simulink model "SecRwRtStLgrstUpwdDnwdIsPosChk"  (R2024b)
settings: Solver=FixedStepDiscrete  StartTime=0.0  StopTime=10.0  FixedStep=0.01  RelTol=1e-3
undefined symbols (not defined in the file or in its folder): KeSMSuSecRwStLegrestUpwdDwnwdPosDelta_Val, KeSMSuSecRwStLegrestUpwdDwnwdPosTolr_Val
libraries: StIsPosChkLib x19, simulink x8
(part 1 of 2)
settings Model: Creator=sn2xws  LastModifiedBy=sn55gm
settings Model: ModifiedHistory=|
  | 2023.8.1 V2.0.0 CR421790 增加模式21-26
  | 2024.7.8 V3.0.0 557模式流程V1.9
  | 2024.8.15 V3.0.1 智享模式需要计算目标位置，不能直接判断到位置，posalready赋值0
  | 2024.9.5 V3.0.2 新增Md56，注释不用的模式
  | 2024.10.14 V3.0.3 新增Md57 Md58
  | 2024.11.27 V3.0.4 Md57运行时不能直接判断到位置
  | 25.7.7 V3.13.0 新增Md61 Md62 md30 md31
  | 25.7.15 Md30secstage2done_Val_read增加接口作为目标位置判断
settings SolverCC: AlgebraicLoopSolver=TrustRegion
settings DataIOCC: SaveFormat=StructureWithTime  ReturnWorkspaceOutputs=off
settings OptimizationCC: DefaultParameterBehavior=Inlined  EnhancedBackFolding=on  PassReuseOutputArgsAs=Individual arguments  ZeroExternalMemoryAtStartup=off  ZeroInternalMemoryAtStartup=off  OptimizeBlockOrder=speed  DifferentSizesBufferReuse=on  OptimizationCustomize=off  EfficientTunableParamExpr=on
settings DebuggingCC: ParameterTunabilityLossMsg=error  UnconnectedInputMsg=warning  UnconnectedOutputMsg=warning  UnconnectedLineMsg=warning  ArithmeticOperatorsInVariantConditions=warning
settings ModelReferenceCC: EnableRefExpFcnMdlSchedulingChecks=on  ModelReferenceNumInstancesAllowed=Single
settings SFSimCC: MATLABDynamicMemAlloc=off  CustomCodeUndefinedFunction=UseInterfaceOnly
settings RTWCC: Description=AUTOSAR  SystemTargetFile=autosar.tlc  GenCodeOnly=on  TemplateMakefile=ert_default_tmf  GenerateReport=on  IncludeHyperlinkInReport=on  LaunchReport=on  DataTypeReplacement=CDataTypesFixedWidth  GenerateTraceInfo=on  GenerateTraceReport=on  GenerateTraceReportSl=on  GenerateTraceReportSf=on  GenerateTraceReportEml=on  GPUComputeCapability=3.5
settings CodeAppCC: ForceParamTrailComments=on  IgnoreCustomStorageClasses=off  OperatorAnnotations=on  SimulinkDataObjDesc=on  SFDataObjDesc=on  InsertBlockDesc=on
settings STFCustomTargetCC: TargetLangStandard=C99 (ISO)  MultiwordLength=256  ParMdlRefBuildCompliant=on  CompOptLevelCompliant=on  IncludeMdlTerminateFcn=off  CombineOutputUpdateFcns=on  SuppressErrorStatus=on  ERTCustomFileBanners=on  SupportNonFinite=off  SupportComplex=off  SupportContinuousTime=off  SupportNonInlinedSFcns=off  RemoveResetFunc=on  MATLABClassNameForMDSCustomization=Simulink.SoftwareTarget.ERTCustomization  AutosarCompliant=on  UseToolchainInfoCompliant=on  LookupTableObjectStructAxisOrder=2,1,3,4,...  LUTObjectStructOrderEvenSpacing=Size,Table,Breakpoints  SystemTargetFile=autosar.tlc
settings ERTTargetCC: TargetLangStandard=C99 (ISO)  ConcurrentExecutionCompliant=off  IncludeMdlTerminateFcn=off  SuppressErrorStatus=on  SupportNonFinite=off  SupportComplex=off  ModelStepFunctionPrototypeControlCompliant=off  CPPClassGenCompliant=off  AutosarCompliant=on  LookupTableObjectStructAxisOrder=2,1,3,4,...  LUTObjectStructOrderEvenSpacing=Size,Table,Breakpoints  ERTCustomFileTemplate=example_file_process.tlc  ERTFilePackagingFormat=Compact  BooleanTrueId=TRUE  BooleanFalseId=FALSE  DynamicArrayContainerType=coder::array

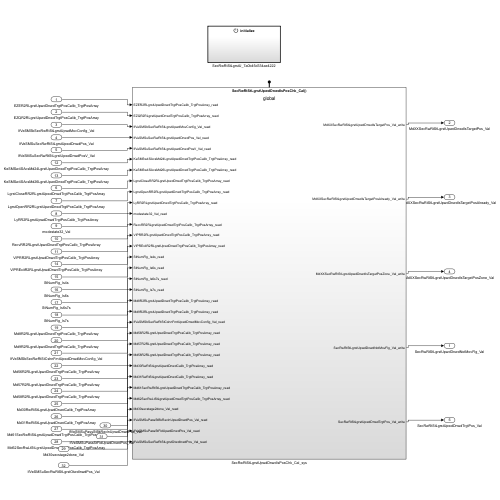
[thumbnail: Simulink's stored preview of the top-level diagram]
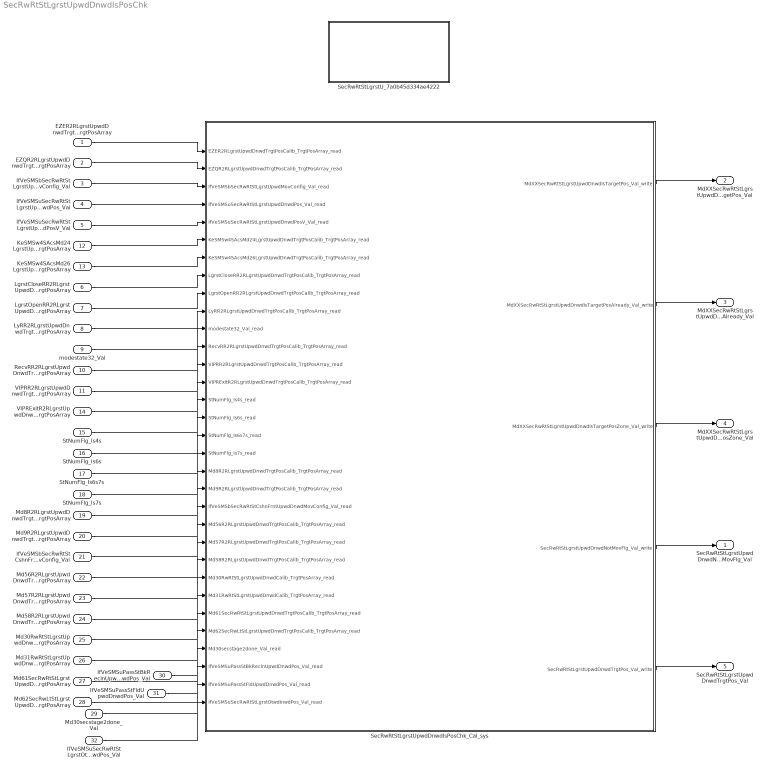
== system SecRwRtStLgrstUpwdDnwdIsPosChk ==
  EZER2RLgrstUpwdDnwdTrgtPosCalib_TrgtPosArray : Inport  Description=|  OutDataTypeStr=uint16  PortDimensions=3
      | 0:Pos
      | 1:Max
      | 2:Min
  EZQR2RLgrstUpwdDnwdTrgtPosCalib_TrgtPosArray : Inport  Description=|  Port=2  OutDataTypeStr=uint16  PortDimensions=3
      | 0:Pos
      | 1:Max
      | 2:Min
  IfVeSMSbSecRwRtStLgrstUpwdMovConfig_Val : Inport  Port=3  OutDataTypeStr=boolean  PortDimensions=1
  IfVeSMSuSecRwRtStLgrstUpwdDnwdPos_Val : Inport  Port=4  OutDataTypeStr=uint16  PortDimensions=1
  IfVeSMSuSecRwRtStLgrstUpwdDnwdPosV_Val : Inport  Port=5  OutDataTypeStr=boolean  PortDimensions=1
  LgrstCloseRR2RLgrstUpwdDnwdTrgtPosCalib_TrgtPosArray : Inport  Description=|  Port=6  OutDataTypeStr=uint16  PortDimensions=3
      | 0:Pos
      | 1:Max
      | 2:Min
  LgrstOpenRR2RLgrstUpwdDnwdTrgtPosCalib_TrgtPosArray : Inport  Description=|  Port=7  OutDataTypeStr=uint16  PortDimensions=3
      | 0:Pos
      | 1:Max
      | 2:Min
  LyRR2RLgrstUpwdDnwdTrgtPosCalib_TrgtPosArray : Inport  Description=|  Port=8  OutDataTypeStr=uint16  PortDimensions=3
      | 0:Pos
      | 1:Max
      | 2:Min
  modestate32_Val : Inport  Port=9  OutDataTypeStr=uint32  PortDimensions=1
  RecvRR2RLgrstUpwdDnwdTrgtPosCalib_TrgtPosArray : Inport  Description=|  Port=10  OutDataTypeStr=uint16  PortDimensions=3
      | 0:Pos
      | 1:Max
      | 2:Min
  VIPRR2RLgrstUpwdDnwdTrgtPosCalib_TrgtPosArray : Inport  Description=|  Port=11  OutDataTypeStr=uint16  PortDimensions=3
      | 0:Pos
      | 1:Max
      | 2:Min
  KeSMSw4SAcsMd24LgrstUpwdDnwdTrgtPosCalib_TrgtPosArray : Inport  Description=|  Port=12  OutDataTypeStr=uint16  PortDimensions=3
      | 0:Pos
      | 1:Max
      | 2:Min
  KeSMSw4SAcsMd26LgrstUpwdDnwdTrgtPosCalib_TrgtPosArray : Inport  Description=|  Port=13  OutDataTypeStr=uint16  PortDimensions=3
      | 0:Pos
      | 1:Max
      | 2:Min
  VIPRExitR2RLgrstUpwdDnwdTrgtPosCalib_TrgtPosArray : Inport  Description=|  Port=14  OutDataTypeStr=uint16  PortDimensions=3
      | 0:Pos
      | 1:Max
      | 2:Min
  StNumFlg_Is4s : Inport  Port=15  OutDataTypeStr=boolean  PortDimensions=1
  StNumFlg_Is6s : Inport  Port=16  OutDataTypeStr=boolean  PortDimensions=1
  StNumFlg_Is6s7s : Inport  Port=17  OutDataTypeStr=boolean  PortDimensions=1
  StNumFlg_Is7s : Inport  Port=18  OutDataTypeStr=boolean  PortDimensions=1
  Md8R2RLgrstUpwdDnwdTrgtPosCalib_TrgtPosArray : Inport  Description=|  Port=19  OutDataTypeStr=uint16  PortDimensions=3
      | 0:Pos
      | 1:Max
      | 2:Min
  Md9R2RLgrstUpwdDnwdTrgtPosCalib_TrgtPosArray : Inport  Description=|  Port=20  OutDataTypeStr=uint16  PortDimensions=3
      | 0:Pos
      | 1:Max
      | 2:Min
  IfVeSMSbSecRwRtStCshnFrntUpwdDnwdMovConfig_Val : Inport  Port=21  OutDataTypeStr=boolean  PortDimensions=1
  Md56R2RLgrstUpwdDnwdTrgtPosCalib_TrgtPosArray : Inport  Description=|  Port=22  OutDataTypeStr=uint16  PortDimensions=3
      | 0:Pos
      | 1:Max
      | 2:Min
  Md57R2RLgrstUpwdDnwdTrgtPosCalib_TrgtPosArray : Inport  Description=|  Port=23  OutDataTypeStr=uint16  PortDimensions=3
      | 0:Pos
      | 1:Max
      | 2:Min
  Md58R2RLgrstUpwdDnwdTrgtPosCalib_TrgtPosArray : Inport  Description=|  Port=24  OutDataTypeStr=uint16  PortDimensions=3
      | 0:Pos
      | 1:Max
      | 2:Min
  Md30RwRtStLgrstUpwdDnwdCalib_TrgtPosArray : Inport  Description=|  Port=25  OutDataTypeStr=uint16  PortDimensions=3
      | 0:Pos
      | 1:Max
      | 2:Min
  Md31RwRtStLgrstUpwdDnwdCalib_TrgtPosArray : Inport  Description=|  Port=26  OutDataTypeStr=uint16  PortDimensions=3
      | 0:Pos
      | 1:Max
      | 2:Min
  Md61SecRwRtStLgrstUpwdDnwdTrgtPosCalib_TrgtPosArray : Inport  Description=|  Port=27  OutDataTypeStr=uint16  PortDimensions=3
      | 0:Pos
      | 1:Max
      | 2:Min
  Md62SecRwLtStLgrstUpwdDnwdTrgtPosCalib_TrgtPosArray : Inport  Description=|  Port=28  OutDataTypeStr=uint16  PortDimensions=3
      | 0:Pos
      | 1:Max
      | 2:Min
  Md30secstage2done_Val : Inport  Port=29  OutDataTypeStr=uint8  PortDimensions=1
  IfVeSMSuPassStBkReclnUpwdDnwdPos_Val : Inport  Port=30  OutDataTypeStr=uint16  PortDimensions=1
  IfVeSMSuPassStFldUpwdDnwdPos_Val : Inport  Port=31  OutDataTypeStr=uint16  PortDimensions=1
  IfVeSMSuSecRwRtStLgrstOtwdInwdPos_Val : Inport  Port=32  OutDataTypeStr=uint16  PortDimensions=1
  SecRwRtStLgrstU_7a0b45d334ae4222 : Subsystem
  SecRwRtStLgrstUpwdDnwdIsPosChk_Cal_sys : Subsystem
  SecRwRtStLgrstUpwdDnwdNotMovFlg_Val : Outport  OutDataTypeStr=boolean  PortDimensions=1  VectorParamsAs1DForOutWhenUnconnected=off
  MdXXSecRwRtStLgrstUpwdDnwdIsTargetPos_Val : Outport  Port=2  OutDataTypeStr=uint32  PortDimensions=1  VectorParamsAs1DForOutWhenUnconnected=off
  MdXXSecRwRtStLgrstUpwdDnwdIsTargetPosAlready_Val : Outport  Port=3  OutDataTypeStr=uint32  PortDimensions=1  VectorParamsAs1DForOutWhenUnconnected=off
  MdXXSecRwRtStLgrstUpwdDnwdIsTargetPosZone_Val : Outport  Port=4  OutDataTypeStr=uint32  PortDimensions=1  VectorParamsAs1DForOutWhenUnconnected=off
  SecRwRtStLgrstUpwdDnwdTrgtPos_Val : Outport  Port=5  OutDataTypeStr=uint16  PortDimensions=1  VectorParamsAs1DForOutWhenUnconnected=off
  wires:
  EZER2RLgrstUpwdDnwdTrgtPosCalib_TrgtPosArray/1 -> SecRwRtStLgrstUpwdDnwdIsPosChk_Cal_sys/1(EZER2RLgrstUpwdDnwdTrgtPosCalib_TrgtPosArray_read)
  EZQR2RLgrstUpwdDnwdTrgtPosCalib_TrgtPosArray/1 -> SecRwRtStLgrstUpwdDnwdIsPosChk_Cal_sys/2(EZQR2RLgrstUpwdDnwdTrgtPosCalib_TrgtPosArray_read)
  IfVeSMSbSecRwRtStLgrstUpwdMovConfig_Val/1 -> SecRwRtStLgrstUpwdDnwdIsPosChk_Cal_sys/3(IfVeSMSbSecRwRtStLgrstUpwdMovConfig_Val_read)
  IfVeSMSuSecRwRtStLgrstUpwdDnwdPos_Val/1 -> SecRwRtStLgrstUpwdDnwdIsPosChk_Cal_sys/4(IfVeSMSuSecRwRtStLgrstUpwdDnwdPos_Val_read)
  IfVeSMSuSecRwRtStLgrstUpwdDnwdPosV_Val/1 -> SecRwRtStLgrstUpwdDnwdIsPosChk_Cal_sys/5(IfVeSMSuSecRwRtStLgrstUpwdDnwdPosV_Val_read)
  LgrstCloseRR2RLgrstUpwdDnwdTrgtPosCalib_TrgtPosArray/1 -> SecRwRtStLgrstUpwdDnwdIsPosChk_Cal_sys/8(LgrstCloseRR2RLgrstUpwdDnwdTrgtPosCalib_TrgtPosArray_read)
  LgrstOpenRR2RLgrstUpwdDnwdTrgtPosCalib_TrgtPosArray/1 -> SecRwRtStLgrstUpwdDnwdIsPosChk_Cal_sys/9(LgrstOpenRR2RLgrstUpwdDnwdTrgtPosCalib_TrgtPosArray_read)
  LyRR2RLgrstUpwdDnwdTrgtPosCalib_TrgtPosArray/1 -> SecRwRtStLgrstUpwdDnwdIsPosChk_Cal_sys/10(LyRR2RLgrstUpwdDnwdTrgtPosCalib_TrgtPosArray_read)
  modestate32_Val/1 -> SecRwRtStLgrstUpwdDnwdIsPosChk_Cal_sys/11(modestate32_Val_read)
  RecvRR2RLgrstUpwdDnwdTrgtPosCalib_TrgtPosArray/1 -> SecRwRtStLgrstUpwdDnwdIsPosChk_Cal_sys/12(RecvRR2RLgrstUpwdDnwdTrgtPosCalib_TrgtPosArray_read)
  VIPRR2RLgrstUpwdDnwdTrgtPosCalib_TrgtPosArray/1 -> SecRwRtStLgrstUpwdDnwdIsPosChk_Cal_sys/13(VIPRR2RLgrstUpwdDnwdTrgtPosCalib_TrgtPosArray_read)
  SecRwRtStLgrstUpwdDnwdIsPosChk_Cal_sys/1(MdXXSecRwRtStLgrstUpwdDnwdIsTargetPos_Val_write) -> MdXXSecRwRtStLgrstUpwdDnwdIsTargetPos_Val/1
  SecRwRtStLgrstUpwdDnwdIsPosChk_Cal_sys/2(MdXXSecRwRtStLgrstUpwdDnwdIsTargetPosAlready_Val_write) -> MdXXSecRwRtStLgrstUpwdDnwdIsTargetPosAlready_Val/1
  SecRwRtStLgrstUpwdDnwdIsPosChk_Cal_sys/3(MdXXSecRwRtStLgrstUpwdDnwdIsTargetPosZone_Val_write) -> MdXXSecRwRtStLgrstUpwdDnwdIsTargetPosZone_Val/1
  SecRwRtStLgrstUpwdDnwdIsPosChk_Cal_sys/4(SecRwRtStLgrstUpwdDnwdNotMovFlg_Val_write) -> SecRwRtStLgrstUpwdDnwdNotMovFlg_Val/1
  SecRwRtStLgrstUpwdDnwdIsPosChk_Cal_sys/5(SecRwRtStLgrstUpwdDnwdTrgtPos_Val_write) -> SecRwRtStLgrstUpwdDnwdTrgtPos_Val/1
  KeSMSw4SAcsMd24LgrstUpwdDnwdTrgtPosCalib_TrgtPosArray/1 -> SecRwRtStLgrstUpwdDnwdIsPosChk_Cal_sys/6(KeSMSw4SAcsMd24LgrstUpwdDnwdTrgtPosCalib_TrgtPosArray_read)
  KeSMSw4SAcsMd26LgrstUpwdDnwdTrgtPosCalib_TrgtPosArray/1 -> SecRwRtStLgrstUpwdDnwdIsPosChk_Cal_sys/7(KeSMSw4SAcsMd26LgrstUpwdDnwdTrgtPosCalib_TrgtPosArray_read)
  VIPRExitR2RLgrstUpwdDnwdTrgtPosCalib_TrgtPosArray/1 -> SecRwRtStLgrstUpwdDnwdIsPosChk_Cal_sys/14(VIPRExitR2RLgrstUpwdDnwdTrgtPosCalib_TrgtPosArray_read)
  StNumFlg_Is4s/1 -> SecRwRtStLgrstUpwdDnwdIsPosChk_Cal_sys/15(StNumFlg_Is4s_read)
  StNumFlg_Is6s/1 -> SecRwRtStLgrstUpwdDnwdIsPosChk_Cal_sys/16(StNumFlg_Is6s_read)
  StNumFlg_Is6s7s/1 -> SecRwRtStLgrstUpwdDnwdIsPosChk_Cal_sys/17(StNumFlg_Is6s7s_read)
  StNumFlg_Is7s/1 -> SecRwRtStLgrstUpwdDnwdIsPosChk_Cal_sys/18(StNumFlg_Is7s_read)
  Md8R2RLgrstUpwdDnwdTrgtPosCalib_TrgtPosArray/1 -> SecRwRtStLgrstUpwdDnwdIsPosChk_Cal_sys/19(Md8R2RLgrstUpwdDnwdTrgtPosCalib_TrgtPosArray_read)
  Md9R2RLgrstUpwdDnwdTrgtPosCalib_TrgtPosArray/1 -> SecRwRtStLgrstUpwdDnwdIsPosChk_Cal_sys/20(Md9R2RLgrstUpwdDnwdTrgtPosCalib_TrgtPosArray_read)
  IfVeSMSbSecRwRtStCshnFrntUpwdDnwdMovConfig_Val/1 -> SecRwRtStLgrstUpwdDnwdIsPosChk_Cal_sys/21(IfVeSMSbSecRwRtStCshnFrntUpwdDnwdMovConfig_Val_read)
  Md56R2RLgrstUpwdDnwdTrgtPosCalib_TrgtPosArray/1 -> SecRwRtStLgrstUpwdDnwdIsPosChk_Cal_sys/22(Md56R2RLgrstUpwdDnwdTrgtPosCalib_TrgtPosArray_read)
  Md57R2RLgrstUpwdDnwdTrgtPosCalib_TrgtPosArray/1 -> SecRwRtStLgrstUpwdDnwdIsPosChk_Cal_sys/23(Md57R2RLgrstUpwdDnwdTrgtPosCalib_TrgtPosArray_read)
  Md58R2RLgrstUpwdDnwdTrgtPosCalib_TrgtPosArray/1 -> SecRwRtStLgrstUpwdDnwdIsPosChk_Cal_sys/24(Md58R2RLgrstUpwdDnwdTrgtPosCalib_TrgtPosArray_read)
  Md30RwRtStLgrstUpwdDnwdCalib_TrgtPosArray/1 -> SecRwRtStLgrstUpwdDnwdIsPosChk_Cal_sys/25(Md30RwRtStLgrstUpwdDnwdCalib_TrgtPosArray_read)
  Md31RwRtStLgrstUpwdDnwdCalib_TrgtPosArray/1 -> SecRwRtStLgrstUpwdDnwdIsPosChk_Cal_sys/26(Md31RwRtStLgrstUpwdDnwdCalib_TrgtPosArray_read)
  Md61SecRwRtStLgrstUpwdDnwdTrgtPosCalib_TrgtPosArray/1 -> SecRwRtStLgrstUpwdDnwdIsPosChk_Cal_sys/27(Md61SecRwRtStLgrstUpwdDnwdTrgtPosCalib_TrgtPosArray_read)
  Md62SecRwLtStLgrstUpwdDnwdTrgtPosCalib_TrgtPosArray/1 -> SecRwRtStLgrstUpwdDnwdIsPosChk_Cal_sys/28(Md62SecRwLtStLgrstUpwdDnwdTrgtPosCalib_TrgtPosArray_read)
  Md30secstage2done_Val/1 -> SecRwRtStLgrstUpwdDnwdIsPosChk_Cal_sys/29(Md30secstage2done_Val_read)
  IfVeSMSuPassStBkReclnUpwdDnwdPos_Val/1 -> SecRwRtStLgrstUpwdDnwdIsPosChk_Cal_sys/30(IfVeSMSuPassStBkReclnUpwdDnwdPos_Val_read)
  IfVeSMSuPassStFldUpwdDnwdPos_Val/1 -> SecRwRtStLgrstUpwdDnwdIsPosChk_Cal_sys/31(IfVeSMSuPassStFldUpwdDnwdPos_Val_read)
  IfVeSMSuSecRwRtStLgrstOtwdInwdPos_Val/1 -> SecRwRtStLgrstUpwdDnwdIsPosChk_Cal_sys/32(IfVeSMSuSecRwRtStLgrstOtwdInwdPos_Val_read)

== system SecRwRtStLgrstUpwdDnwdIsPosChk/SecRwRtStLgrstU_7a0b45d334ae4222 ==
  note: Added blocks
  note: Added blocks
  Event Listener : EventListener  EventName=reset
  PA_KeSMSuSecRwStLegrestUpwdDwnwdPosDelta_Val : Constant  Value=KeSMSuSecRwStLegrestUpwdDwnwdPosDelta_Val
  PA_KeSMSuSecRwStLegrestUpwdDwnwdPosTolr_Val : Constant  Value=KeSMSuSecRwStLegrestUpwdDwnwdPosTolr_Val
  Terminator_1 : Terminator
  Terminator_2 : Terminator
  wires:
  PA_KeSMSuSecRwStLegrestUpwdDwnwdPosDelta_Val/1 -> Terminator_1/1
  PA_KeSMSuSecRwStLegrestUpwdDwnwdPosTolr_Val/1 -> Terminator_2/1

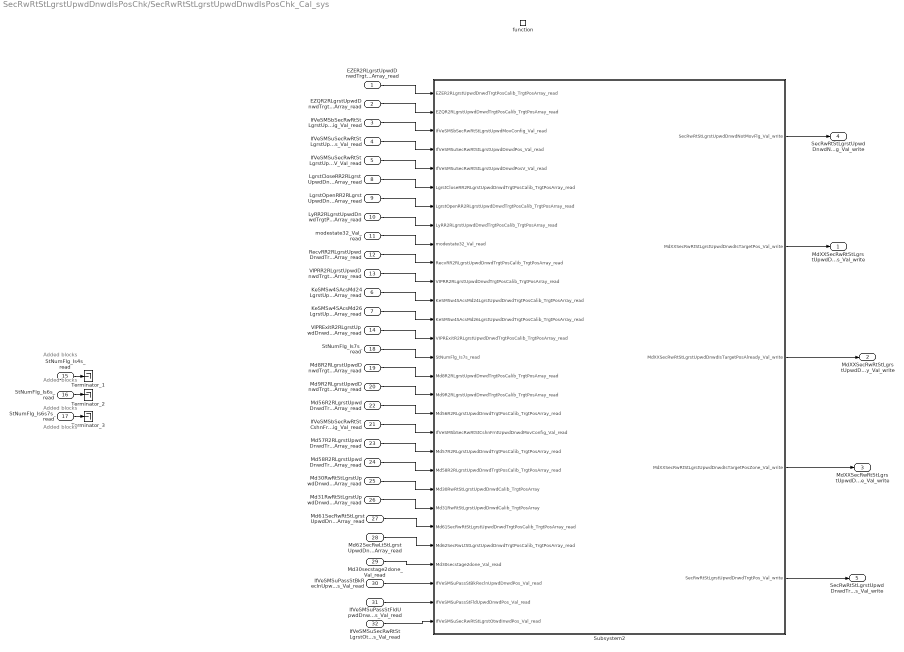
== system SecRwRtStLgrstUpwdDnwdIsPosChk/SecRwRtStLgrstUpwdDnwdIsPosChk_Cal_sys ==
  note: Added blocks
  note: Added blocks
  note: Added blocks
  note: Added blocks
  EZER2RLgrstUpwdDnwdTrgtPosCalib_TrgtPosArray_read : Inport
  EZQR2RLgrstUpwdDnwdTrgtPosCalib_TrgtPosArray_read : Inport  Port=2
  IfVeSMSbSecRwRtStLgrstUpwdMovConfig_Val_read : Inport  Port=3
  IfVeSMSuSecRwRtStLgrstUpwdDnwdPos_Val_read : Inport  Port=4
  IfVeSMSuSecRwRtStLgrstUpwdDnwdPosV_Val_read : Inport  Port=5
  KeSMSw4SAcsMd24LgrstUpwdDnwdTrgtPosCalib_TrgtPosArray_read : Inport  Port=6
  KeSMSw4SAcsMd26LgrstUpwdDnwdTrgtPosCalib_TrgtPosArray_read : Inport  Port=7
  LgrstCloseRR2RLgrstUpwdDnwdTrgtPosCalib_TrgtPosArray_read : Inport  Port=8
  LgrstOpenRR2RLgrstUpwdDnwdTrgtPosCalib_TrgtPosArray_read : Inport  Port=9
  LyRR2RLgrstUpwdDnwdTrgtPosCalib_TrgtPosArray_read : Inport  Port=10
  modestate32_Val_read : Inport  Port=11
  RecvRR2RLgrstUpwdDnwdTrgtPosCalib_TrgtPosArray_read : Inport  Port=12
  VIPRR2RLgrstUpwdDnwdTrgtPosCalib_TrgtPosArray_read : Inport  Port=13
  VIPRExitR2RLgrstUpwdDnwdTrgtPosCalib_TrgtPosArray_read : Inport  Port=14
  StNumFlg_Is4s_read : Inport  Port=15
  StNumFlg_Is6s_read : Inport  Port=16
  StNumFlg_Is6s7s_read : Inport  Port=17
  StNumFlg_Is7s_read : Inport  Port=18
  Md8R2RLgrstUpwdDnwdTrgtPosCalib_TrgtPosArray_read : Inport  Port=19
  Md9R2RLgrstUpwdDnwdTrgtPosCalib_TrgtPosArray_read : Inport  Port=20
  IfVeSMSbSecRwRtStCshnFrntUpwdDnwdMovConfig_Val_read : Inport  Port=21
  Md56R2RLgrstUpwdDnwdTrgtPosCalib_TrgtPosArray_read : Inport  Port=22
  Md57R2RLgrstUpwdDnwdTrgtPosCalib_TrgtPosArray_read : Inport  Port=23
  Md58R2RLgrstUpwdDnwdTrgtPosCalib_TrgtPosArray_read : Inport  Port=24
  Md30RwRtStLgrstUpwdDnwdCalib_TrgtPosArray_read : Inport  Port=25
  Md31RwRtStLgrstUpwdDnwdCalib_TrgtPosArray_read : Inport  Port=26
  Md61SecRwRtStLgrstUpwdDnwdTrgtPosCalib_TrgtPosArray_read : Inport  Port=27
  Md62SecRwLtStLgrstUpwdDnwdTrgtPosCalib_TrgtPosArray_read : Inport  Port=28
  Md30secstage2done_Val_read : Inport  Port=29
  IfVeSMSuPassStBkReclnUpwdDnwdPos_Val_read : Inport  Port=30
  IfVeSMSuPassStFldUpwdDnwdPos_Val_read : Inport  Port=31
  IfVeSMSuSecRwRtStLgrstOtwdInwdPos_Val_read : Inport  Port=32
  function : TriggerPort  TriggerType=function-call  IsSimulinkFunction=on  FunctionName=SecRwRtStLgrstUpwdDnwdIsPosChk_Cal  VariantControl=(inherit)
  Subsystem2 : Subsystem
  Terminator_1 : Terminator
  Terminator_2 : Terminator
  Terminator_3 : Terminator
  MdXXSecRwRtStLgrstUpwdDnwdIsTargetPos_Val_write : Outport  VectorParamsAs1DForOutWhenUnconnected=off
      settings: EnsureOutportIsVirtual=on
  MdXXSecRwRtStLgrstUpwdDnwdIsTargetPosAlready_Val_write : Outport  Port=2  VectorParamsAs1DForOutWhenUnconnected=off
      settings: EnsureOutportIsVirtual=on
  MdXXSecRwRtStLgrstUpwdDnwdIsTargetPosZone_Val_write : Outport  Port=3  VectorParamsAs1DForOutWhenUnconnected=off
      settings: EnsureOutportIsVirtual=on
  SecRwRtStLgrstUpwdDnwdNotMovFlg_Val_write : Outport  Port=4  VectorParamsAs1DForOutWhenUnconnected=off
      settings: EnsureOutportIsVirtual=on
  SecRwRtStLgrstUpwdDnwdTrgtPos_Val_write : Outport  Port=5  VectorParamsAs1DForOutWhenUnconnected=off
      settings: EnsureOutportIsVirtual=on
  wires:
  EZER2RLgrstUpwdDnwdTrgtPosCalib_TrgtPosArray_read/1 -> Subsystem2/1(EZER2RLgrstUpwdDnwdTrgtPosCalib_TrgtPosArray_read)
  EZQR2RLgrstUpwdDnwdTrgtPosCalib_TrgtPosArray_read/1 -> Subsystem2/2(EZQR2RLgrstUpwdDnwdTrgtPosCalib_TrgtPosArray_read)
  IfVeSMSbSecRwRtStLgrstUpwdMovConfig_Val_read/1 -> Subsystem2/3(IfVeSMSbSecRwRtStLgrstUpwdMovConfig_Val_read)
  IfVeSMSuSecRwRtStLgrstUpwdDnwdPos_Val_read/1 -> Subsystem2/4(IfVeSMSuSecRwRtStLgrstUpwdDnwdPos_Val_read)
  IfVeSMSuSecRwRtStLgrstUpwdDnwdPosV_Val_read/1 -> Subsystem2/5(IfVeSMSuSecRwRtStLgrstUpwdDnwdPosV_Val_read)
  LgrstCloseRR2RLgrstUpwdDnwdTrgtPosCalib_TrgtPosArray_read/1 -> Subsystem2/6(LgrstCloseRR2RLgrstUpwdDnwdTrgtPosCalib_TrgtPosArray_read)
  LgrstOpenRR2RLgrstUpwdDnwdTrgtPosCalib_TrgtPosArray_read/1 -> Subsystem2/7(LgrstOpenRR2RLgrstUpwdDnwdTrgtPosCalib_TrgtPosArray_read)
  LyRR2RLgrstUpwdDnwdTrgtPosCalib_TrgtPosArray_read/1 -> Subsystem2/8(LyRR2RLgrstUpwdDnwdTrgtPosCalib_TrgtPosArray_read)
  modestate32_Val_read/1 -> Subsystem2/9(modestate32_Val_read)
  RecvRR2RLgrstUpwdDnwdTrgtPosCalib_TrgtPosArray_read/1 -> Subsystem2/10(RecvRR2RLgrstUpwdDnwdTrgtPosCalib_TrgtPosArray_read)
  VIPRR2RLgrstUpwdDnwdTrgtPosCalib_TrgtPosArray_read/1 -> Subsystem2/11(VIPRR2RLgrstUpwdDnwdTrgtPosCalib_TrgtPosArray_read)
  KeSMSw4SAcsMd24LgrstUpwdDnwdTrgtPosCalib_TrgtPosArray_read/1 -> Subsystem2/12(KeSMSw4SAcsMd24LgrstUpwdDnwdTrgtPosCalib_TrgtPosArray_read)
  KeSMSw4SAcsMd26LgrstUpwdDnwdTrgtPosCalib_TrgtPosArray_read/1 -> Subsystem2/13(KeSMSw4SAcsMd26LgrstUpwdDnwdTrgtPosCalib_TrgtPosArray_read)
  Subsystem2/1(SecRwRtStLgrstUpwdDnwdNotMovFlg_Val_write) -> SecRwRtStLgrstUpwdDnwdNotMovFlg_Val_write/1
  Subsystem2/2(MdXXSecRwRtStLgrstUpwdDnwdIsTargetPos_Val_write) -> MdXXSecRwRtStLgrstUpwdDnwdIsTargetPos_Val_write/1
  Subsystem2/3(MdXXSecRwRtStLgrstUpwdDnwdIsTargetPosAlready_Val_write) -> MdXXSecRwRtStLgrstUpwdDnwdIsTargetPosAlready_Val_write/1
  Subsystem2/5(SecRwRtStLgrstUpwdDnwdTrgtPos_Val_write) -> SecRwRtStLgrstUpwdDnwdTrgtPos_Val_write/1
  Subsystem2/4(MdXXSecRwRtStLgrstUpwdDnwdIsTargetPosZone_Val_write) -> MdXXSecRwRtStLgrstUpwdDnwdIsTargetPosZone_Val_write/1
  VIPRExitR2RLgrstUpwdDnwdTrgtPosCalib_TrgtPosArray_read/1 -> Subsystem2/14(VIPRExitR2RLgrstUpwdDnwdTrgtPosCalib_TrgtPosArray_read)
  StNumFlg_Is4s_read/1 -> Terminator_1/1
  StNumFlg_Is6s_read/1 -> Terminator_2/1
  StNumFlg_Is6s7s_read/1 -> Terminator_3/1
  StNumFlg_Is7s_read/1 -> Subsystem2/15(StNumFlg_Is7s_read)
  Md8R2RLgrstUpwdDnwdTrgtPosCalib_TrgtPosArray_read/1 -> Subsystem2/16(Md8R2RLgrstUpwdDnwdTrgtPosCalib_TrgtPosArray_read)
  Md9R2RLgrstUpwdDnwdTrgtPosCalib_TrgtPosArray_read/1 -> Subsystem2/17(Md9R2RLgrstUpwdDnwdTrgtPosCalib_TrgtPosArray_read)
  Md56R2RLgrstUpwdDnwdTrgtPosCalib_TrgtPosArray_read/1 -> Subsystem2/18(Md56R2RLgrstUpwdDnwdTrgtPosCalib_TrgtPosArray_read)
  IfVeSMSbSecRwRtStCshnFrntUpwdDnwdMovConfig_Val_read/1 -> Subsystem2/19(IfVeSMSbSecRwRtStCshnFrntUpwdDnwdMovConfig_Val_read)
  Md57R2RLgrstUpwdDnwdTrgtPosCalib_TrgtPosArray_read/1 -> Subsystem2/20(Md57R2RLgrstUpwdDnwdTrgtPosCalib_TrgtPosArray_read)
  Md58R2RLgrstUpwdDnwdTrgtPosCalib_TrgtPosArray_read/1 -> Subsystem2/21(Md58R2RLgrstUpwdDnwdTrgtPosCalib_TrgtPosArray_read)
  Md30RwRtStLgrstUpwdDnwdCalib_TrgtPosArray_read/1 -> Subsystem2/22(Md30RwRtStLgrstUpwdDnwdCalib_TrgtPosArray)
  Md31RwRtStLgrstUpwdDnwdCalib_TrgtPosArray_read/1 -> Subsystem2/23(Md31RwRtStLgrstUpwdDnwdCalib_TrgtPosArray)
  Md61SecRwRtStLgrstUpwdDnwdTrgtPosCalib_TrgtPosArray_read/1 -> Subsystem2/24(Md61SecRwRtStLgrstUpwdDnwdTrgtPosCalib_TrgtPosArray_read)
  Md62SecRwLtStLgrstUpwdDnwdTrgtPosCalib_TrgtPosArray_read/1 -> Subsystem2/25(Md62SecRwLtStLgrstUpwdDnwdTrgtPosCalib_TrgtPosArray_read)
  Md30secstage2done_Val_read/1 -> Subsystem2/26(Md30secstage2done_Val_read)
  IfVeSMSuPassStBkReclnUpwdDnwdPos_Val_read/1 -> Subsystem2/27(IfVeSMSuPassStBkReclnUpwdDnwdPos_Val_read)
  IfVeSMSuPassStFldUpwdDnwdPos_Val_read/1 -> Subsystem2/28(IfVeSMSuPassStFldUpwdDnwdPos_Val_read)
  IfVeSMSuSecRwRtStLgrstOtwdInwdPos_Val_read/1 -> Subsystem2/29(IfVeSMSuSecRwRtStLgrstOtwdInwdPos_Val_read)

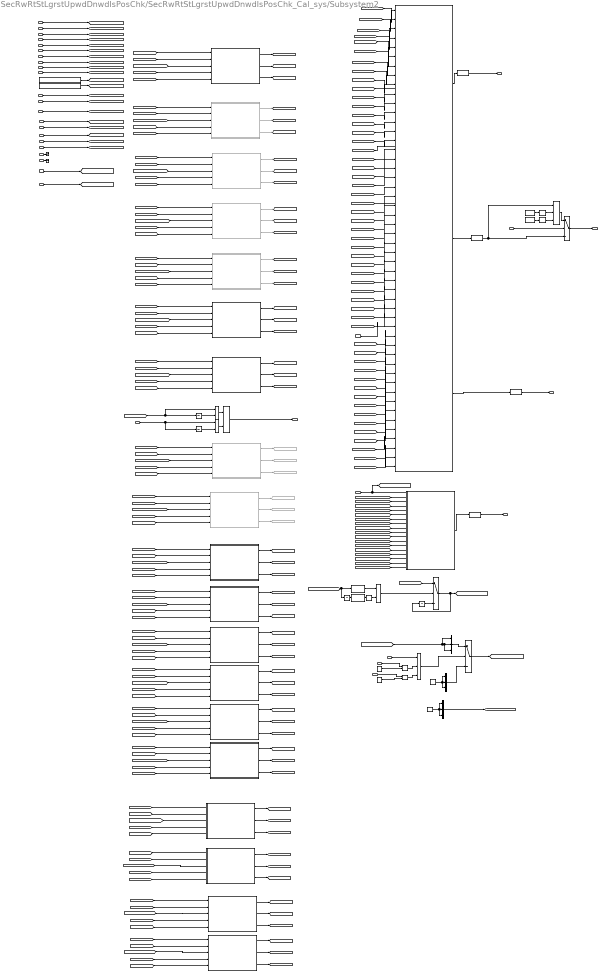
== system SecRwRtStLgrstUpwdDnwdIsPosChk/SecRwRtStLgrstUpwdDnwdIsPosChk_Cal_sys/Subsystem2 ==
  note: 2023.8.1 V2.0.0 CR421790 增加模式21-26
  EZER2RLgrstUpwdDnwdTrgtPosCalib_TrgtPosArray_read : Inport
  EZQR2RLgrstUpwdDnwdTrgtPosCalib_TrgtPosArray_read : Inport  Port=2
  IfVeSMSbSecRwRtStLgrstUpwdMovConfig_Val_read : Inport  Port=3
  IfVeSMSuSecRwRtStLgrstUpwdDnwdPos_Val_read : Inport  Port=4
  IfVeSMSuSecRwRtStLgrstUpwdDnwdPosV_Val_read : Inport  Port=5
  LgrstCloseRR2RLgrstUpwdDnwdTrgtPosCalib_TrgtPosArray_read : Inport  Port=6
  LgrstOpenRR2RLgrstUpwdDnwdTrgtPosCalib_TrgtPosArray_read : Inport  Port=7
  LyRR2RLgrstUpwdDnwdTrgtPosCalib_TrgtPosArray_read : Inport  Port=8
  modestate32_Val_read : Inport  Port=9
  RecvRR2RLgrstUpwdDnwdTrgtPosCalib_TrgtPosArray_read : Inport  Port=10
  VIPRR2RLgrstUpwdDnwdTrgtPosCalib_TrgtPosArray_read : Inport  Port=11
  KeSMSw4SAcsMd24LgrstUpwdDnwdTrgtPosCalib_TrgtPosArray_read : Inport  Port=12
  KeSMSw4SAcsMd26LgrstUpwdDnwdTrgtPosCalib_TrgtPosArray_read : Inport  Port=13
  VIPRExitR2RLgrstUpwdDnwdTrgtPosCalib_TrgtPosArray_read : Inport  Port=14
  StNumFlg_Is7s_read : Inport  Port=15
  Md8R2RLgrstUpwdDnwdTrgtPosCalib_TrgtPosArray_read : Inport  Port=16
  Md9R2RLgrstUpwdDnwdTrgtPosCalib_TrgtPosArray_read : Inport  Port=17
  Md56R2RLgrstUpwdDnwdTrgtPosCalib_TrgtPosArray_read : Inport  Port=18
  IfVeSMSbSecRwRtStCshnFrntUpwdDnwdMovConfig_Val_read : Inport  Port=19
  Md57R2RLgrstUpwdDnwdTrgtPosCalib_TrgtPosArray_read : Inport  Port=20
  Md58R2RLgrstUpwdDnwdTrgtPosCalib_TrgtPosArray_read : Inport  Port=21
  Md30RwRtStLgrstUpwdDnwdCalib_TrgtPosArray : Inport  Port=22
  Md31RwRtStLgrstUpwdDnwdCalib_TrgtPosArray : Inport  Port=23
  Md61SecRwRtStLgrstUpwdDnwdTrgtPosCalib_TrgtPosArray_read : Inport  Port=24
  Md62SecRwLtStLgrstUpwdDnwdTrgtPosCalib_TrgtPosArray_read : Inport  Port=25
  Md30secstage2done_Val_read : Inport  Port=26
  IfVeSMSuPassStBkReclnUpwdDnwdPos_Val_read : Inport  Port=27
  IfVeSMSuPassStFldUpwdDnwdPos_Val_read : Inport  Port=28
  IfVeSMSuSecRwRtStLgrstOtwdInwdPos_Val_read : Inport  Port=29
  32BitSelector1 : StIsPosChkLib/32BitSelector  BitNum=29
  32BitSelector14 : StIsPosChkLib/32BitSelector  BitNum=29
  Bitwise Operator : simulink/Logic and Bit Operations/Bitwise Operator  logicop=AND  UseBitMask=off  NumInputPorts=3  BitMask=bin2dec('11011001')  BitMaskRealWorld=Stored Integer
  Bitwise Operator1 : simulink/Logic and Bit Operations/Bitwise Operator  logicop=NOT  UseBitMask=off  BitMask=bin2dec('11011001')  BitMaskRealWorld=Stored Integer
  Bitwise Operator2 : simulink/Logic and Bit Operations/Bitwise Operator  logicop=NOT  UseBitMask=off  BitMask=bin2dec('11011001')  BitMaskRealWorld=Stored Integer
  Constant : Constant  Value=2048  OutDataTypeStr=uint32
  Constant1 : Constant  Value=1048576  OutDataTypeStr=uint32
  Constant10 : Constant  Value=0  OutDataTypeStr=uint16
  Constant2 : Constant  Value=120
  Constant3 : Constant  Value=120
  Constant9 : Constant  Value=0  OutDataTypeStr=uint16
  Data Type Conversion{,1..3} (4 alike) : DataTypeConversion  SaturateOnIntegerOverflow=off  RndMeth=Floor
  Goto36 : Goto  Commented=on  GotoTag=Md24IsTargetPosAlready
  Goto37 : Goto  Commented=on  GotoTag=Md24IsTargetPos
  Goto38 : Goto  Commented=on  GotoTag=Md24IsTargetPosZone
  Goto39 : Goto  Commented=on  GotoTag=Md26IsTargetPosAlready
  Goto40 : Goto  Commented=on  GotoTag=Md26IsTargetPos
  Goto41 : Goto  Commented=on  GotoTag=Md26IsTargetPosZone
  Logical Operator : Logic  AllPortsSameDT=off  OutDataTypeStr=boolean
  Logical Operator1 : Logic  Operator=NOT  AllPortsSameDT=off  OutDataTypeStr=boolean
  Logical Operator2 : Logic  Inputs=3  AllPortsSameDT=off  OutDataTypeStr=boolean
  Logical Operator3 : Logic  AllPortsSameDT=off  OutDataTypeStr=boolean
  Mux1 : Mux  Inputs=3
  Mux6 : Mux  Inputs=3
  Mux7 : Mux  Inputs=3
  PA_KeSMSuSecRwStLegrestUpwdDwnwdPosDelta_Val : Constant  Value=KeSMSuSecRwStLegrestUpwdDwnwdPosDelta_Val
  PA_KeSMSuSecRwStLegrestUpwdDwnwdPosTolr_Val : Constant  Value=KeSMSuSecRwStLegrestUpwdDwnwdPosTolr_Val
  Relational Operator : RelationalOperator  Operator=<=  OutDataTypeStr=boolean  RndMeth=Simplest  InputSameDT=off
  Relational Operator1 : RelationalOperator  Operator=<=  OutDataTypeStr=boolean  RndMeth=Simplest  InputSameDT=off
  Relational Operator2 : RelationalOperator  Operator===  OutDataTypeStr=boolean  RndMeth=Simplest  InputSameDT=off
  Relational Operator3 : RelationalOperator  Operator===  OutDataTypeStr=boolean  RndMeth=Simplest  InputSameDT=off
  Subsystem : Subsystem
  Subsystem1 : Subsystem
  Subsystem10 : Subsystem  Commented=on
  Subsystem11 : Subsystem
  Subsystem12 : Subsystem
  Subsystem13 : Subsystem
  Subsystem14 : Subsystem
  Subsystem15 : Subsystem
  Subsystem16 : Subsystem
  Subsystem17 : Subsystem
  Subsystem18 : Subsystem
  Subsystem19 : Subsystem
  Subsystem2 : Subsystem
  Subsystem20 : Subsystem
  Subsystem3 : Subsystem  Commented=on
  Subsystem4 : Subsystem  Commented=on
  Subsystem5 : Subsystem  Commented=on
  Subsystem6 : Subsystem  Commented=on
  Subsystem7 : Subsystem
  Subsystem8 : Subsystem
  Subsystem9 : Subsystem  Commented=on
  Switch : Switch  Criteria=u2 > Threshold  SaturateOnIntegerOverflow=off  InputSameDT=off
  Switch2 : Switch  Criteria=u2 > Threshold  SaturateOnIntegerOverflow=off  InputSameDT=off
  Switch3 : Switch  Criteria=u2 > Threshold  SaturateOnIntegerOverflow=off  InputSameDT=off
  Terminator_1 : Terminator
  Terminator_2 : Terminator
  Unit Delay{,1..3} (4 alike) : UnitDelay  SampleTime=-1  HasFrameUpgradeWarning=on
  SecRwRtStLgrstUpwdDnwdNotMovFlg_Val_write : Outport  VectorParamsAs1DForOutWhenUnconnected=off
      settings: EnsureOutportIsVirtual=on
  MdXXSecRwRtStLgrstUpwdDnwdIsTargetPos_Val_write : Outport  Port=2  VectorParamsAs1DForOutWhenUnconnected=off
      settings: EnsureOutportIsVirtual=on
  MdXXSecRwRtStLgrstUpwdDnwdIsTargetPosAlready_Val_write : Outport  Port=3  VectorParamsAs1DForOutWhenUnconnected=off
      settings: EnsureOutportIsVirtual=on
  MdXXSecRwRtStLgrstUpwdDnwdIsTargetPosZone_Val_write : Outport  Port=4  VectorParamsAs1DForOutWhenUnconnected=off
      settings: EnsureOutportIsVirtual=on
  SecRwRtStLgrstUpwdDnwdTrgtPos_Val_write : Outport  Port=5  VectorParamsAs1DForOutWhenUnconnected=off
      settings: EnsureOutportIsVirtual=on
  wires:
  [EZECalib] -> Subsystem2/3(CalibArray)
  [PosDelta] -> Subsystem6/4(Delta)
  Subsystem5/1(IsPos) -> [LgrstCloseLIsTargetPos]
  [LgrstOpenLCalib] -> Subsystem/2(LgrstOpenLCalib)
  RecvRR2RLgrstUpwdDnwdTrgtPosCalib_TrgtPosArray_read/1 -> [RecvLCalib]
  VIPRR2RLgrstUpwdDnwdTrgtPosCalib_TrgtPosArray_read/1 -> [VIPLCalib]
  [Pos] -> Subsystem6/2(Pos)
  Subsystem6/3(IsPosAlready) -> [LyLIsTargetPosAlready]
  [RecvLIsTargetPosAlready] -> Subsystem1/16(RecvLIsTargetPosAlready)
  [Pos] -> Subsystem7/2(Pos)
  PA_KeSMSuSecRwStLegrestUpwdDwnwdPosDelta_Val/1 -> [PosDelta]
  IfVeSMSuSecRwRtStLgrstUpwdDnwdPos_Val_read/1 -> [Pos]
  [VIPLIsTargetPosZone] -> Subsystem1/23(VIPLIsTargetPosZone)
  [PosDelta] -> Subsystem8/4(Delta)
  [PosTolr] -> Subsystem4/5(Tolr)
  [PosV] -> Subsystem6/1(PosV)
  Subsystem8/3(IsPosAlready) -> [VIPLIsTargetPosAlready]
  [LgrstOpenLIsTargetPosAlready] -> Subsystem1/14(LgrstOpenLIsTargetPosAlready)
  Data Type Conversion/1 -> SecRwRtStLgrstUpwdDnwdTrgtPos_Val_write/1
  [EZQIsTargetPosAlready] -> Subsystem1/19(EZQIsTargetPosAlready)
  Subsystem4/3(IsPosAlready) -> [LgrstOpenLIsTargetPosAlready]
  [LyLCalib] -> Subsystem6/3(CalibArray)
  [PosV] -> Subsystem7/1(PosV)
  Subsystem4/1(IsPos) -> [LgrstOpenLIsTargetPos]
  [RecvLCalib] -> Subsystem7/3(CalibArray)
  [EZEIsTargetPos] -> Subsystem1/12(EZEIsTargetPos)
  [Pos] -> Subsystem3/2(Pos)
  Subsystem7/1(IsPos) -> [RecvLIsTargetPos]
  Subsystem7/2(IsPosZone) -> [RecvLIsTargetPosZone]
  Subsystem2/1(IsPos) -> [EZEIsTargetPos]
  [PosDelta] -> Subsystem2/4(Delta)
  Subsystem2/2(IsPosZone) -> [EZEIsTargetPosZone]
  [PosTolr] -> Subsystem7/5(Tolr)
  Subsystem8/1(IsPos) -> [VIPLIsTargetPos]
  [PosV] -> Subsystem2/1(PosV)
  [EZEIsTargetPosZone] -> Subsystem1/24(EZEIsTargetPosZone)
  IfVeSMSuSecRwRtStLgrstUpwdDnwdPosV_Val_read/1 -> [PosV]
  [LyLIsTargetPos] -> ?
  Subsystem4/2(IsPosZone) -> [LgrstOpenLIsTargetPosZone]
  PA_KeSMSuSecRwStLegrestUpwdDwnwdPosTolr_Val/1 -> [PosTolr]
  Subsystem8/2(IsPosZone) -> [VIPLIsTargetPosZone]
  [PosV] -> Subsystem4/1(PosV)
  LyRR2RLgrstUpwdDnwdTrgtPosCalib_TrgtPosArray_read/1 -> [LyLCalib]
  [EZQCalib] -> Subsystem3/3(CalibArray)
  LgrstOpenRR2RLgrstUpwdDnwdTrgtPosCalib_TrgtPosArray_read/1 -> [LgrstOpenLCalib]
  [LgrstCloseLIsTargetPos] -> Subsystem1/9(LgrstCloseLIsTargetPos)
  Subsystem3/2(IsPosZone) -> [EZQIsTargetPosZone]
  LgrstCloseRR2RLgrstUpwdDnwdTrgtPosCalib_TrgtPosArray_read/1 -> [LgrstCloseLCalib]
  Subsystem3/3(IsPosAlready) -> [EZQIsTargetPosAlready]
  [Pos] -> Subsystem4/2(Pos)
  Subsystem2/3(IsPosAlready) -> [EZEIsTargetPosAlready]
  Subsystem1/3(IsTargetPosZone) -> Data Type Conversion3/1
  [PosTolr] -> Subsystem8/5(Tolr)
  [VIPLCalib] -> Subsystem/6(VIPLCalib)
  EZER2RLgrstUpwdDnwdTrgtPosCalib_TrgtPosArray_read/1 -> [EZECalib]
  [EZQCalib] -> Subsystem/8(EZQCalib)
  [LgrstCloseLIsTargetPosAlready] -> Subsystem1/15(LgrstCloseLIsTargetPosAlready)
  [EZQIsTargetPosZone] -> Subsystem1/25(EZQIsTargetPosZone)
  Subsystem6/2(IsPosZone) -> [LyLIsTargetPosZone]
  [RecvLIsTargetPosZone] -> Subsystem1/22(RecvLIsTargetPosZone)
  Subsystem3/1(IsPos) -> [EZQIsTargetPos]
  [LgrstOpenLIsTargetPos] -> Subsystem1/8(LgrstOpenLIsTargetPos)
  [VIPLIsTargetPos] -> Subsystem1/11(VIPLIsTargetPos)
  Logical Operator3/1 -> SecRwRtStLgrstUpwdDnwdNotMovFlg_Val_write/1
  [Pos] -> Subsystem8/2(Pos)
  [PosV] -> Subsystem3/1(PosV)
  [VIPLCalib] -> Subsystem8/3(CalibArray)
  modestate32_Val_read/1 -> [modestate32_Val_read], Subsystem/1(modestate32_Val_read)
  [PosDelta] -> Subsystem4/4(Delta)
  Subsystem6/1(IsPos) -> [LyLIsTargetPos]
  [PosTolr] -> Subsystem5/5(Tolr)
  [PosV] -> Subsystem8/1(PosV)
  [MovConfig] -> Subsystem1/7(MovConfig)
  [PosDelta] -> Subsystem5/4(Delta)
  Subsystem5/3(IsPosAlready) -> [LgrstCloseLIsTargetPosAlready]
  Subsystem/1(TrgtPos) -> Data Type Conversion/1
  [RecvLCalib] -> Subsystem/5(RecvLCalib)
  [EZQIsTargetPos] -> Subsystem1/13(EZQIsTargetPos)
  [EZECalib] -> Subsystem/7(EZECalib)
  [PosDelta] -> Subsystem3/4(Delta)
  [PosTolr] -> Subsystem3/5(Tolr)
  [PosTolr] -> Subsystem6/5(Tolr)
  EZQR2RLgrstUpwdDnwdTrgtPosCalib_TrgtPosArray_read/1 -> [EZQCalib]
  [Pos] -> Subsystem2/2(Pos)
  [LyLIsTargetPosAlready] -> ?
  Data Type Conversion3/1 -> MdXXSecRwRtStLgrstUpwdDnwdIsTargetPosZone_Val_write/1
  [VIPLIsTargetPosAlready] -> Subsystem1/17(VIPLIsTargetPosAlready)
  [RecvLIsTargetPos] -> Subsystem1/10(RecvLIsTargetPos)
  [PosDelta] -> Subsystem7/4(Delta)
  Subsystem5/2(IsPosZone) -> [LgrstCloseLIsTargetPosZone]
  [LyLCalib] -> Subsystem/4(LyLCalib)
  [LgrstCloseLIsTargetPosZone] -> Subsystem1/21(LgrstCloseLIsTargetPosZone)
  [EZEIsTargetPosAlready] -> Subsystem1/18(EZEIsTargetPosAlready)
  [PosV] -> Subsystem5/1(PosV)
  [Pos] -> Subsystem5/2(Pos)
  [LyLIsTargetPosZone] -> ?
  Data Type Conversion1/1 -> MdXXSecRwRtStLgrstUpwdDnwdIsTargetPos_Val_write/1
  [LgrstOpenLIsTargetPosZone] -> Subsystem1/20(LgrstOpenLIsTargetPosZone)
  [PosTolr] -> Subsystem2/5(Tolr)
  [LgrstCloseLCalib] -> Subsystem/3(LgrstCloseLCalib)
  Subsystem7/3(IsPosAlready) -> [RecvLIsTargetPosAlready]
  Subsystem1/2(IsTargetPosAlready) -> Data Type Conversion2/1
  Subsystem1/1(IsTargetPos) -> Data Type Conversion1/1
  IfVeSMSbSecRwRtStLgrstUpwdMovConfig_Val_read/1 -> [MovConfig]
  KeSMSw4SAcsMd24LgrstUpwdDnwdTrgtPosCalib_TrgtPosArray_read/1 -> [Md24Calib]
  KeSMSw4SAcsMd26LgrstUpwdDnwdTrgtPosCalib_TrgtPosArray_read/1 -> [Md26Calib]
  [PosV] -> Subsystem9/1(PosV)
  [Md24Calib] -> Subsystem9/3(CalibArray)
  [Pos] -> Subsystem9/2(Pos)
  [PosTolr] -> Subsystem9/5(Tolr)
  Subsystem9/2(IsPosZone) -> Goto38/1
  Subsystem9/1(IsPos) -> Goto37/1
  Subsystem9/3(IsPosAlready) -> Goto36/1
  [PosDelta] -> Subsystem9/4(Delta)
  [PosDelta] -> Subsystem10/4(Delta)
  Subsystem10/3(IsPosAlready) -> Goto39/1
  Subsystem10/1(IsPos) -> Goto40/1
  Subsystem10/2(IsPosZone) -> Goto41/1
  [PosTolr] -> Subsystem10/5(Tolr)
  [Pos] -> Subsystem10/2(Pos)
  [Md26Calib] -> Subsystem10/3(CalibArray)
  [PosV] -> Subsystem10/1(PosV)
  [Md57Calib] -> Subsystem/9(Md57Calib)
  [Md58Calib] -> Subsystem/10(Md58Calib)
  [Md57IsTargetPos] -> Subsystem1/26(Md57IsTargetPos)
  [Md58IsTargetPos] -> Subsystem1/27(Md58IsTargetPos)
  [Md57IsTargetPosAlready] -> Subsystem1/28(Md57IsTargetPosAlready)
  [Md57IsTargetPosZone] -> Subsystem1/30(Md57IsTargetPosZone)
  [Md58IsTargetPosAlready] -> Subsystem1/29(Md58IsTargetPosAlready)
  [Md58IsTargetPosZone] -> Subsystem1/31(Md58IsTargetPosZone)
  [LgrstCloseLCalib] -> Subsystem5/3(CalibArray)
  [LgrstOpenLCalib] -> Subsystem4/3(CalibArray)
  VIPRExitR2RLgrstUpwdDnwdTrgtPosCalib_TrgtPosArray_read/1 -> [Md28Calib]
  [PosV] -> Subsystem11/1(PosV)
  [Md28Calib] -> Subsystem11/3(CalibArray)
  [Pos] -> Subsystem11/2(Pos)
  [PosTolr] -> Subsystem11/5(Tolr)
  Subsystem11/2(IsPosZone) -> [Md28IsTargetPosZone]
  Subsystem11/1(IsPos) -> [Md28IsTargetPos]
  Subsystem11/3(IsPosAlready) -> [Md28IsTargetPosAlready]
  [PosDelta] -> Subsystem11/4(Delta)
  [Md28Calib] -> Subsystem/11(Md28Calib)
  [Md28IsTargetPos] -> Subsystem1/32(Md28IsTargetPos)
  [Md28IsTargetPosAlready] -> Subsystem1/33(Md28IsTargetPosAlready)
  [Md28IsTargetPosZone] -> Subsystem1/34(Md28IsTargetPosZone)
  StNumFlg_Is7s_read/1 -> Subsystem1/35(StNumFlg_Is7s_read)
  Md8R2RLgrstUpwdDnwdTrgtPosCalib_TrgtPosArray_read/1 -> [Md8Calib]
  Md9R2RLgrstUpwdDnwdTrgtPosCalib_TrgtPosArray_read/1 -> [Md9Calib]
  Md56R2RLgrstUpwdDnwdTrgtPosCalib_TrgtPosArray_read/1 -> [Md56Calib]
  [PosDelta] -> Subsystem12/4(Delta)
  Subsystem12/3(IsPosAlready) -> [Md8IsTargetPosAlready]
  Subsystem12/1(IsPos) -> [Md8IsTargetPos]
  Subsystem12/2(IsPosZone) -> [Md8IsTargetPosZone]
  [PosTolr] -> Subsystem12/5(Tolr)
  [Pos] -> Subsystem12/2(Pos)
  [Md8Calib] -> Subsystem12/3(CalibArray)
  [PosV] -> Subsystem12/1(PosV)
  [PosV] -> Subsystem13/1(PosV)
  [Md9Calib] -> Subsystem13/3(CalibArray)
  [Pos] -> Subsystem13/2(Pos)
  [PosTolr] -> Subsystem13/5(Tolr)
  Subsystem13/2(IsPosZone) -> [Md9IsTargetPosZone]
  Subsystem13/1(IsPos) -> [Md9IsTargetPos]
  Subsystem13/3(IsPosAlready) -> [Md9IsTargetPosAlready]
  [PosDelta] -> Subsystem13/4(Delta)
  [PosDelta] -> Subsystem14/4(Delta)
  Subsystem14/3(IsPosAlready) -> [Md56IsTargetPosAlready]
  Subsystem14/1(IsPos) -> [Md56IsTargetPos]
  Subsystem14/2(IsPosZone) -> [Md56IsTargetPosZone]
  [PosTolr] -> Subsystem14/5(Tolr)
  [Pos] -> Subsystem14/2(Pos)
  [Md56Calib] -> Subsystem14/3(CalibArray)
  [PosV] -> Subsystem14/1(PosV)
  [Md56Calib] -> Subsystem/14(Md56Calib)
  [Md9Calib] -> Subsystem/13(Md9Calib)
  [Md8Calib] -> Subsystem/12(Md8Calib)
  [Md8IsTargetPos] -> Subsystem1/36(Md8IsTargetPos)
  [Md9IsTargetPos] -> Subsystem1/37(Md9IsTargetPos)
  [Md56IsTargetPos] -> Subsystem1/38(Md56IsTargetPos)
  [Md8IsTargetPosAlready] -> Subsystem1/39(Md8IsTargetPosAlready)
  [Md9IsTargetPosAlready] -> Subsystem1/40(Md9IsTargetPosAlready)
  [Md56IsTargetPosAlready] -> Subsystem1/41(Md56IsTargetPosAlready)
  [Md8IsTargetPosZone] -> Subsystem1/42(Md8IsTargetPosZone)
  [Md9IsTargetPosZone] -> Subsystem1/43(Md9IsTargetPosZone)
  [Md56IsTargetPosZone] -> Subsystem1/44(Md56IsTargetPosZone)
  Bitwise Operator/1 -> Switch/1
  Bitwise Operator1/1 -> Bitwise Operator/2
  Data Type Conversion2/1 -> Bitwise Operator/1, Switch/3
  Constant/1 -> Bitwise Operator1/1
  Switch/1 -> MdXXSecRwRtStLgrstUpwdDnwdIsTargetPosAlready_Val_write/1
  IfVeSMSbSecRwRtStCshnFrntUpwdDnwdMovConfig_Val_read/1 -> Switch/2
  Md57R2RLgrstUpwdDnwdTrgtPosCalib_TrgtPosArray_read/1 -> [Md57Calib]
  Md58R2RLgrstUpwdDnwdTrgtPosCalib_TrgtPosArray_read/1 -> [Md58Calib]
  [PosV] -> Subsystem15/1(PosV)
  [Md57Calib] -> Subsystem15/3(CalibArray)
  [Pos] -> Subsystem15/2(Pos)
  [PosTolr] -> Subsystem15/5(Tolr)
  Subsystem15/2(IsPosZone) -> [Md57IsTargetPosZone]
  Subsystem15/1(IsPos) -> [Md57IsTargetPos]
  Subsystem15/3(IsPosAlready) -> [Md57IsTargetPosAlready]
  [PosDelta] -> Subsystem15/4(Delta)
  [PosDelta] -> Subsystem16/4(Delta)
  Subsystem16/3(IsPosAlready) -> [Md58IsTargetPosAlready]
  Subsystem16/1(IsPos) -> [Md58IsTargetPos]
  Subsystem16/2(IsPosZone) -> [Md58IsTargetPosZone]
  [PosTolr] -> Subsystem16/5(Tolr)
  [Pos] -> Subsystem16/2(Pos)
  [Md58Calib] -> Subsystem16/3(CalibArray)
  [PosV] -> Subsystem16/1(PosV)
  Bitwise Operator2/1 -> Bitwise Operator/3
  Constant1/1 -> Bitwise Operator2/1
  Subsystem17/1(IsPos) -> [Md30IsTargetPos]
  [PosV] -> Subsystem17/1(PosV)
  [PosDelta] -> Subsystem17/4(Delta)
  [Pos] -> Subsystem17/2(Pos)
  [PosTolr] -> Subsystem17/5(Tolr)
  Subsystem17/3(IsPosAlready) -> [Md30IsTargetPosAlready]
  [Md30calib] -> Subsystem17/3(CalibArray)
  Subsystem17/2(IsPosZone) -> [Md30IsTargetPosZone]
  [PosV] -> Subsystem18/1(PosV)
  [Md31calib] -> Subsystem18/3(CalibArray)
  [PosTolr] -> Subsystem18/5(Tolr)
  [Pos] -> Subsystem18/2(Pos)
  Subsystem18/3(IsPosAlready) -> [Md31IsTargetPosAlready]
  [PosDelta] -> Subsystem18/4(Delta)
  Subsystem18/2(IsPosZone) -> [Md31IsTargetPosZone]
  Subsystem18/1(IsPos) -> [Md31IsTargetPos]
  [Md31IsTargetPosAlready] -> Subsystem1/6(Md31IsTargetPosAlready)
  [Md31IsTargetPosZone] -> Subsystem1/5(Md31IsTargetPosZone)
  [Md31IsTargetPos] -> Subsystem1/4(Md31IsTargetPos)
  [Md30IsTargetPosAlready] -> Subsystem1/3(Md30IsTargetPosAlready)
  [Md30IsTargetPosZone] -> Subsystem1/2(Md30IsTargetPosZone)
  [Md30IsTargetPos] -> Subsystem1/1(Md30IsTargetPos)
  Subsystem19/1(IsPos) -> [Md61IsTargetPos]
  Subsystem19/2(IsPosZone) -> [Md61IsTargetPosZone]
  [PosDelta] -> Subsystem19/4(Delta)
  Subsystem19/3(IsPosAlready) -> [Md61IsTargetPosAlready]
  [Pos] -> Subsystem19/2(Pos)
  [PosTolr] -> Subsystem19/5(Tolr)
  [Md61calib] -> Subsystem19/3(CalibArray)
  [PosV] -> Subsystem19/1(PosV)
  [PosV] -> Subsystem20/1(PosV)
  [Md62calib] -> Subsystem20/3(CalibArray)
  [PosTolr] -> Subsystem20/5(Tolr)
  [Pos] -> Subsystem20/2(Pos)
  Subsystem20/3(IsPosAlready) -> [Md62IsTargetPosAlready]
  [PosDelta] -> Subsystem20/4(Delta)
  Subsystem20/2(IsPosZone) -> [Md62IsTargetPosZone]
  Subsystem20/1(IsPos) -> [Md62IsTargetPos]
  [Md61IsTargetPos] -> Subsystem1/45(Md61IsTargetPos)
  [Md62IsTargetPos] -> Subsystem1/46(Md62IsTargetPos)
  [Md61IsTargetPosAlready] -> Subsystem1/47(Md61IsTargetPosAlready)
  [Md62IsTargetPosAlready] -> Subsystem1/48(Md62IsTargetPosAlready)
  [Md61IsTargetPosZone] -> Subsystem1/49(Md61IsTargetPosZone)
  [Md62IsTargetPosZone] -> Subsystem1/50(Md62IsTargetPosZone)
  [Md30calib] -> Subsystem/15(Md30Calib)
  [Md31calib] -> Subsystem/16(Md31Calib)
  [Md61calib] -> Subsystem/17(Md61Calib)
  [Md62calib] -> Subsystem/18(Md62Calib)
  Md61SecRwRtStLgrstUpwdDnwdTrgtPosCalib_TrgtPosArray_read/1 -> [Md61calib]
  Md62SecRwLtStLgrstUpwdDnwdTrgtPosCalib_TrgtPosArray_read/1 -> [Md62calib]
  32BitSelector14/1 -> Logical Operator/1
  Logical Operator/1 -> Switch2/2
  Unit Delay/1 -> 32BitSelector1/1
  Logical Operator1/1 -> Logical Operator/2
  32BitSelector1/1 -> Logical Operator1/1
  [modestate32_Val_read] -> Unit Delay/1, 32BitSelector14/1
  [Pos] -> Switch2/1
  Switch2/1 -> Unit Delay1/1, [LgrstupdownPosInit]
  [LgrstupdownPosInit] -> Mux1/2, Mux1/3, Mux1/1
  Switch3/1 -> [Md30calib]
  Constant9/1 -> Mux7/1, Mux7/3, Mux7/2
  Constant10/1 -> Mux6/1, Mux6/3, Mux6/2
  Mux6/1 -> [Md31calib]
  Md30RwRtStLgrstUpwdDnwdCalib_TrgtPosArray/1 -> Terminator_1/1
  Md31RwRtStLgrstUpwdDnwdCalib_TrgtPosArray/1 -> Terminator_2/1
  Unit Delay1/1 -> Switch2/3
  Mux7/1 -> Switch3/3
  Mux1/1 -> Switch3/1
  Md30secstage2done_Val_read/1 -> Logical Operator2/1
  IfVeSMSuPassStBkReclnUpwdDnwdPos_Val_read/1 -> Relational Operator/1
  Constant2/1 -> Relational Operator/2
  Constant3/1 -> Relational Operator1/2
  IfVeSMSuPassStFldUpwdDnwdPos_Val_read/1 -> Relational Operator1/1
  Relational Operator/1 -> Logical Operator2/2
  Relational Operator1/1 -> Logical Operator2/3
  Logical Operator2/1 -> Switch3/2
  IfVeSMSuSecRwRtStLgrstOtwdInwdPos_Val_read/1 -> Unit Delay3/1, Relational Operator3/1
  [Pos] -> Relational Operator2/1, Unit Delay2/1
  Unit Delay3/1 -> Relational Operator3/2
  Unit Delay2/1 -> Relational Operator2/2
  Relational Operator2/1 -> Logical Operator3/1
  Relational Operator3/1 -> Logical Operator3/2

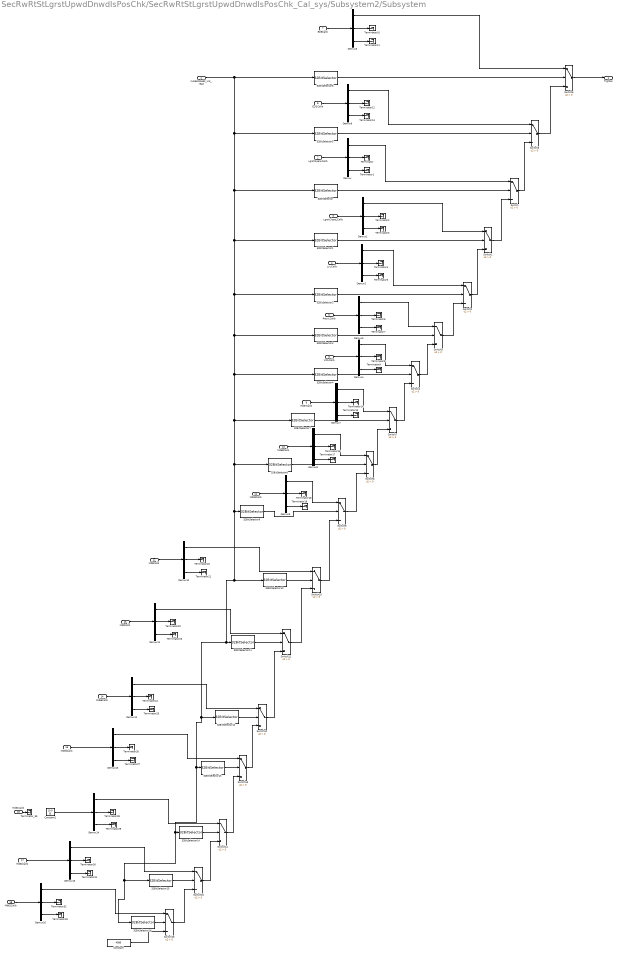
== system SecRwRtStLgrstUpwdDnwdIsPosChk/SecRwRtStLgrstUpwdDnwdIsPosChk_Cal_sys/Subsystem2/Subsystem ==
  modestate32_Val_read : Inport
  LgrstOpenLCalib : Inport  Port=2
  LgrstCloseLCalib : Inport  Port=3
  LyLCalib : Inport  Port=4
  RecvLCalib : Inport  Port=5
  VIPLCalib : Inport  Port=6
  EZECalib : Inport  Port=7
  EZQCalib : Inport  Port=8
  Md57Calib : Inport  Port=9
  Md58Calib : Inport  Port=10
  Md28Calib : Inport  Port=11
  Md8Calib : Inport  Port=12
  Md9Calib : Inport  Port=13
  Md56Calib : Inport  Port=14
  Md30Calib : Inport  Port=15
  Md31Calib : Inport  Port=16
  Md61Calib : Inport  Port=17
  Md62Calib : Inport  Port=18
  32BitSelector : StIsPosChkLib/32BitSelector  BitNum=17
  32BitSelector1 : StIsPosChkLib/32BitSelector  BitNum=18
  32BitSelector10 : StIsPosChkLib/32BitSelector  BitNum=7
  32BitSelector11 : StIsPosChkLib/32BitSelector  BitNum=8
  32BitSelector12 : StIsPosChkLib/32BitSelector  BitNum=24
  32BitSelector13 : StIsPosChkLib/32BitSelector  BitNum=29
  32BitSelector14 : StIsPosChkLib/32BitSelector  BitNum=30
  32BitSelector15 : StIsPosChkLib/32BitSelector  BitNum=5
  32BitSelector16 : StIsPosChkLib/32BitSelector  BitNum=6
  32BitSelector2 : StIsPosChkLib/32BitSelector  BitNum=14
  32BitSelector3 : StIsPosChkLib/32BitSelector  BitNum=12
  32BitSelector4 : StIsPosChkLib/32BitSelector  BitNum=11
  32BitSelector5 : StIsPosChkLib/32BitSelector  BitNum=3
  32BitSelector6 : StIsPosChkLib/32BitSelector  BitNum=0
  32BitSelector7 : StIsPosChkLib/32BitSelector  BitNum=20
  32BitSelector8 : StIsPosChkLib/32BitSelector  BitNum=21
  32BitSelector9 : StIsPosChkLib/32BitSelector  BitNum=27
  Constant : Constant  Value=4095  OutDataTypeStr=uint16
  Constant1 : Constant  Value=[0 0 0]
  Demux{,1..16} (17 alike) : Demux  Outputs=3
  Switch{,1..16} (17 alike) : Switch  Criteria=u2 > Threshold  SaturateOnIntegerOverflow=off  InputSameDT=off
  Terminator{,1..33} (34 alike) : Terminator
  Terminator_35 : Terminator
  TrgtPos : Outport  VectorParamsAs1DForOutWhenUnconnected=off
      settings: EnsureOutportIsVirtual=on
  wires:
  32BitSelector/1 -> Switch/2
  Demux/1 -> Switch/1
  Demux/3 -> Terminator1/1
  Demux/2 -> Terminator/1
  LgrstOpenLCalib/1 -> Demux/1
  LgrstCloseLCalib/1 -> Demux1/1
  Demux1/2 -> Terminator2/1
  Demux1/3 -> Terminator3/1
  Demux1/1 -> Switch1/1
  Switch1/1 -> Switch/3
  32BitSelector1/1 -> Switch1/2
  Switch2/1 -> Switch1/3
  Switch3/1 -> Switch2/3
  Switch4/1 -> Switch3/3
  32BitSelector2/1 -> Switch2/2
  32BitSelector3/1 -> Switch3/2
  32BitSelector4/1 -> Switch4/2
  Demux2/1 -> Switch2/1
  Demux2/3 -> Terminator5/1
  Demux2/2 -> Terminator4/1
  LyLCalib/1 -> Demux2/1
  RecvLCalib/1 -> Demux3/1
  Demux3/2 -> Terminator6/1
  Demux3/3 -> Terminator7/1
  Demux3/1 -> Switch3/1
  Demux4/1 -> Switch4/1
  Demux4/3 -> Terminator9/1
  Demux4/2 -> Terminator8/1
  VIPLCalib/1 -> Demux4/1
  32BitSelector6/1 -> Switch6/2
  Switch5/1 -> Switch6/3
  Switch/1 -> Switch5/3
  Switch6/1 -> TrgtPos/1
  EZECalib/1 -> Demux5/1
  Demux5/2 -> Terminator10/1
  Demux5/3 -> Terminator11/1
  Demux5/1 -> Switch6/1
  32BitSelector5/1 -> Switch5/2
  Demux6/1 -> Switch5/1
  Demux6/3 -> Terminator13/1
  Demux6/2 -> Terminator12/1
  EZQCalib/1 -> Demux6/1
  Md57Calib/1 -> Demux7/1
  Demux7/2 -> Terminator14/1
  Demux7/3 -> Terminator15/1
  Demux7/1 -> Switch7/1
  32BitSelector7/1 -> Switch7/2
  Switch8/1 -> Switch7/3
  32BitSelector8/1 -> Switch8/2
  Demux8/1 -> Switch8/1
  Demux8/3 -> Terminator17/1
  Demux8/2 -> Terminator16/1
  Md58Calib/1 -> Demux8/1
  Switch7/1 -> Switch4/3
  Switch9/1 -> Switch8/3
  Md28Calib/1 -> Demux9/1
  Demux9/2 -> Terminator18/1
  Demux9/3 -> Terminator19/1
  Demux9/1 -> Switch9/1
  32BitSelector9/1 -> Switch9/2
  modestate32_Val_read/1 -> 32BitSelector6/1, 32BitSelector5/1, 32BitSelector/1, 32BitSelector1/1, 32BitSelector2/1, 32BitSelector3/1, 32BitSelector4/1, 32BitSelector10/1, 32BitSelector16/1, 32BitSelector15/1, 32BitSelector14/1, 32BitSelector13/1, 32BitSelector12/1, 32BitSelector11/1, 32BitSelector9/1, 32BitSelector8/1, 32BitSelector7/1
  Switch10/1 -> Switch9/3
  Switch11/1 -> Switch10/3
  Switch12/1 -> Switch11/3
  Demux10/1 -> Switch10/1
  Demux10/3 -> Terminator21/1
  Demux10/2 -> Terminator20/1
  Md8Calib/1 -> Demux10/1
  32BitSelector10/1 -> Switch10/2
  32BitSelector11/1 -> Switch11/2
  32BitSelector12/1 -> Switch12/2
  Md9Calib/1 -> Demux11/1
  Demux11/2 -> Terminator22/1
  Demux11/3 -> Terminator23/1
  Demux11/1 -> Switch11/1
  Demux12/1 -> Switch12/1
  Demux12/3 -> Terminator25/1
  Demux12/2 -> Terminator24/1
  Md56Calib/1 -> Demux12/1
  Switch13/1 -> Switch12/3
  32BitSelector13/1 -> Switch13/2
  Switch14/1 -> Switch13/3
  32BitSelector14/1 -> Switch14/2
  Switch15/1 -> Switch14/3
  Switch16/1 -> Switch15/3
  32BitSelector15/1 -> Switch15/2
  32BitSelector16/1 -> Switch16/2
  Constant/1 -> Switch16/3
  Demux13/2 -> Terminator26/1
  Demux13/3 -> Terminator27/1
  Demux13/1 -> Switch13/1
  Demux14/1 -> Switch14/1
  Demux14/3 -> Terminator29/1
  Demux14/2 -> Terminator28/1
  Demux15/2 -> Terminator30/1
  Demux15/3 -> Terminator31/1
  Demux15/1 -> Switch15/1
  Demux16/1 -> Switch16/1
  Demux16/3 -> Terminator33/1
  Demux16/2 -> Terminator32/1
  Md62Calib/1 -> Demux16/1
  Md30Calib/1 -> Demux13/1
  Md61Calib/1 -> Demux15/1
  Constant1/1 -> Demux14/1
  Md31Calib/1 -> Terminator_35/1
